simulink model "test_control_model_simulation"  (R2019b)
settings: Solver=VariableStepAuto  StartTime=0.0  StopTime=10.0  RelTol=1e-3
settings Model: Creator=a1752760  LastModifiedBy=a1752760

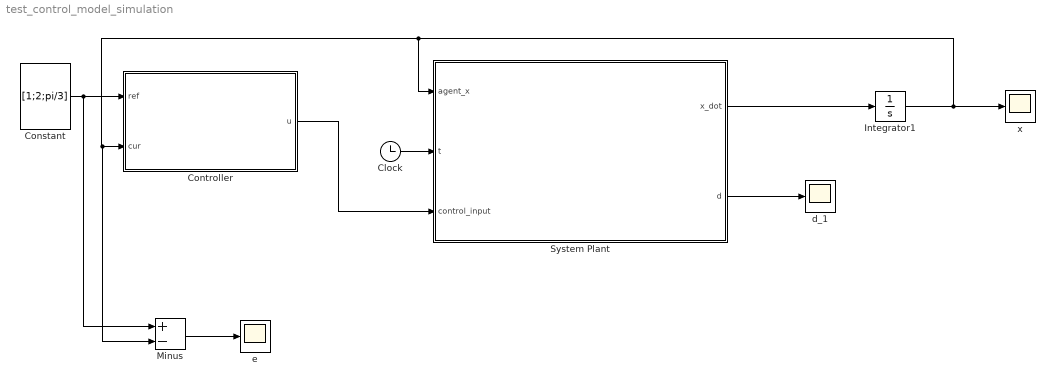
== system test_control_model_simulation ==
  Clock : Clock
  Constant : Constant  Value=[1;2;pi/3]
  Controller : MATLAB Function  TreatAsAtomicUnit=on
  Integrator1 : Integrator  Tag=Position_x1  InitialCondition=[0;0;1/6*pi]  ContinuousStateAttributes='position'
  Minus : Sum  Inputs=+-
  System Plant : MATLAB Function  TreatAsAtomicUnit=on
  d_1 : Scope
  e : Scope
  x : Scope
  wires:
  Integrator1/1 -> System Plant/1(agent_x), Minus/2, Controller/2(cur), x/1
  System Plant/1(x_dot) -> Integrator1/1
  System Plant/2(d) -> d_1/1
  Constant/1 -> Minus/1, Controller/1(ref)
  Clock/1 -> System Plant/2(t)
  Controller/1(u) -> System Plant/3(control_input)
  Minus/1 -> e/1

== matlab function test_control_model_simulation/Controller ==
  data: ref input; u output; cur input
function u = p_controller(ref, cur)



Radius=[0.24;0.23;0.30;0.28;0.25];
serial_num = 1; 
% m=Mass(serial_num);
R=Radius(serial_num);

theta = cur(3);

T = [ -sin(theta), cos(theta), R; 
    -sin(pi/3 - theta), -cos(pi/3 - theta), R;
    sin(pi/3 + theta), -cos(pi/3 + theta), R];

e = ref - cur;
k_p = 5;

u = k_p * T * e;






end

== matlab function test_control_model_simulation/System Plant ==
  data: agent_x input; x_dot output; t input; control_input input; d output
function [x_dot, d] = physical_model( agent_x, t, control_input )

%% Note
% System output
% v_dot: the acceleration vector
% w: the matched disturbances
% saturation status: off
% model is established by the driving force provided by the motor

%% basic parameters set of agents
% Mass=[4.8;4.5;5.5;5.3;5.0];
Radius=[0.24;0.23;0.30;0.28;0.25];
% Inertia=[0.15;0.12;0.25;0.21;0.15];


%% assign the parameter according to serial number
serial_num = 1; 
% m=Mass(serial_num);
R=Radius(serial_num);
% inertia=Inertia(serial_num);


%% current states of the robot
dimension=3;

x=agent_x(1);
y=agent_x(2);
theta=agent_x(dimension);

%% time-varying matched disturbances
% matched_disturbance= [0.5*sin(1.5*t+pi/4*serial_num+x)+2; 0.6*cos(2*t+pi/3*serial_num+0.5*y)+1.5; 0.5*sin(0.8*t+pi/5*serial_num+0.4*theta)+1];

d= [0.3*sin(t)+0.2; 0.1*cos(1.5*t)+0.2; 0.2*sin(1.2*t+pi/3)+0.1];

%% the real model of robot
% M=diag([1/m,1/m,1/inertia]);
T=[-sin(theta), -sin(pi/3-theta), sin(pi/3+theta);
    cos(theta), -cos(pi/3-theta), -cos(pi/3+theta);
    R,          R,                  R];

% fx = -beta*M*(T*T')*agent_v;


g=T;

%% saturation is added here for convinience
% Vmax=6; % the maximum voltage of the motor
% 
% u1up=Vmax/(alpha*m)*(abs(sin(theta))+abs(sin(pi/3-theta))+abs(sin(pi/3+theta)));
% u1do=-Vmax/(alpha*m)*(abs(sin(theta))+abs(sin(pi/3-theta))+abs(sin(pi/3+theta)));
% u2up=Vmax/(alpha*m)*(abs(cos(theta))+abs(cos(pi/3-theta))+abs(cos(pi/3+theta)));
% u2do=-Vmax/(alpha*m)*(abs(cos(theta))+abs(cos(pi/3-theta))+abs(cos(pi/3+theta)));
% u3up=R/(alpha*inertia)*3*Vmax;
% u3do=-R/(alpha*inertia)*3*Vmax;
% 
% control_input(1) = max( min(control_input(1),u1up), u1do );
% control_input(2) = max( min(control_input(2),u2up), u2do );
% control_input(3) = max( min(control_input(3),u3up), u3do );

%% plant output

% w=fx + matched_disturbance; 

d = [0;0;0];

x_dot = d + g* control_input;


end
